simulink model "Temp7"  (R2018b)
settings: Solver=FixedStepAuto  StartTime=0.0  StopTime=10.0  FixedStep=0.01  RelTol=1e-3
settings Model: Creator=mganesan  LastModifiedBy=mganesan
settings OptimizationCC: DefaultParameterBehavior=Inlined  EnhancedBackFolding=on  PassReuseOutputArgsAs=Individual arguments  OptimizeBlockOrder=speed  DifferentSizesBufferReuse=on  OptimizationCustomize=off
settings DebuggingCC: ParameterTunabilityLossMsg=error
settings SFSimCC: SimCustomHeaderCode="#include \"WritePtr.h\""  SimUserSources=WritePtr.c  MATLABDynamicMemAlloc=off
settings RTWCC: SystemTargetFile=ert.tlc  TemplateMakefile=ert_default_tmf  GenerateReport=on  IncludeHyperlinkInReport=on  LaunchReport=on  GenerateTraceInfo=on  GenerateTraceReport=on  GenerateTraceReportSl=on  GenerateTraceReportSf=on  GenerateTraceReportEml=on
settings CodeAppCC: ForceParamTrailComments=on  IgnoreCustomStorageClasses=off  OperatorAnnotations=on  SimulinkDataObjDesc=on  SFDataObjDesc=on  InsertBlockDesc=on
settings ERTTargetCC: TargetLangStandard=C99 (ISO)  GenerateSampleERTMain=on  InlinedParameterPlacement=NonHierarchical  ERTCustomFileTemplate=example_file_process.tlc

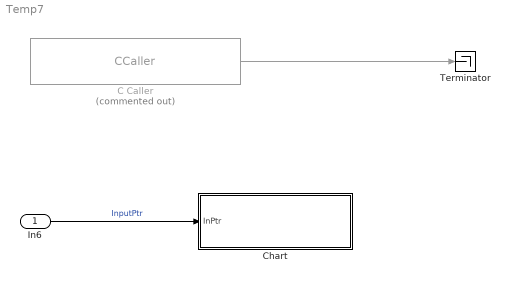
== system Temp7 ==
  In6 : Inport
  C Caller : CCaller  Commented=on  FunctionName=WritePtr  PortSpecificationStruct="%)30     .    Z $   8    (     @         %    \"     $    !     0         %  0 \"0    $    V    07)G3F%M90  4&]R=$YA;64 4V-O<&4     26YD97@     5'EP90      4VEZ90         .    .     8    (    !          %    \"     $    &     0         0    !@   %!T<E9A<@  #@   #@    &    \"     0         !0    @    !    !@    $         $     8   !0=')687(   X    X    !@    @    $          4    (     0    8    !         !     &    3W5T<'5T   .    .     8    (    !@         %    \"     $    !     0         )    \"               #@   #@    &    \"     0         !0    @    !    !0    $         $     4   !U:6YT.     X    P    !@    @    $          4    (     0    (    !         !   @ Q,"
  Chart : Stateflow chart  TreatAsAtomicUnit=on
  Terminator : Terminator
  wires:
  In6/1 -> Chart/1(InPtr)  "InputPtr"
  C Caller/1 -> Terminator/1

== stateflow chart Temp7/Chart ==
  state Init
    en:
    WritePtr(&InPtr);
  (default) -> Init
  data: InPtr input
